simulink model "mpc_CSTR_PQ"  (R2017a)
settings: Solver=ode45  StartTime=0.0  StopTime=5  RelTol=1e-3
values from neighbouring files (symbols this model uses):
  Ap = [-1/(R*C)   1/C        0    -1/C      1/C        0 ... (first row only)    [GeneradoresInterconectados.m]
  Bp = [    0      0 ... (first row only)    [GeneradoresInterconectados.m]
  Cp = [    1      0 ... (first row only)    [GeneradoresInterconectados.m]
  Dp = zeros(2,2)    [GeneradoresInterconectados.m]
  I2 = 18    [GeneradoresInterconectados.m]
  Vabc = 160    [GeneradoresInterconectados.m]
undefined symbols (not defined in the file or in its folder): PI
libraries: powerlib_meascontrol x2, mpclib x1
settings Model: ExtModeTrigMode=oneshot  ExtModeArmWhenConnect=off  Creator=The MathWorks Inc.  LastModifiedBy=MarioAndres
settings DataIOCC: SaveFormat=Array  SaveOutput=off  SignalLogging=off  DSMLogging=off  SaveTime=off  SignalLoggingName=sigsOut
settings OptimizationCC: BooleanDataType=off  ExpressionDepthLimit=2147483647  InitFltsAndDblsToZero=on  LifeSpan=inf
settings DebuggingCC: SaveWithParameterizedLinksMsg=none  UnderspecifiedInitializationDetection=Classic  MergeDetectMultiDrivingBlocksExec=none  SignalResolutionControl=TryResolveAllWithWarning  MultiTaskDSMMsg=warning  MultiTaskCondExecSysMsg=none  IntegerOverflowMsg=none  FcnCallInpInsideContextMsg=warning  StateNameClashWarn=warning  SFUnexpectedBacktrackingDiag=warning  SFNoUnconditionalDefaultTransitionDiag=warning  SFExecutionAtInitializationDiag=none  IntegerSaturationMsg=none
settings HardwareCC: ProdBitPerPointer=32  ProdBitPerSizeT=32  ProdBitPerPtrDiffT=32  ProdLargestAtomicFloat=None  ProdIntDivRoundTo=Undefined  ProdEndianess=Unspecified  ProdWordSize=32  ProdHWDeviceType=32-bit Generic  TargetUnknown=on
settings ModelReferenceCC: PropagateSignalLabelsOutOfModel=off
settings GRTTargetCC: TargetFcnLib=ansi_tfl_tmw.mat  TargetLangStandard=C89/C90 (ANSI)  GeneratePreprocessorConditionals=Disable all  CombineOutputUpdateFcns=off  GRTInterface=on
settings ConfigComp: CovMetricSettings=dw  CovHtmlReporting=on  CovSaveCumulativeToWorkspaceVar=on  CovSaveSingleToWorkspaceVar=on  CovExternalEMLEnable=off  CovSFcnEnable=off

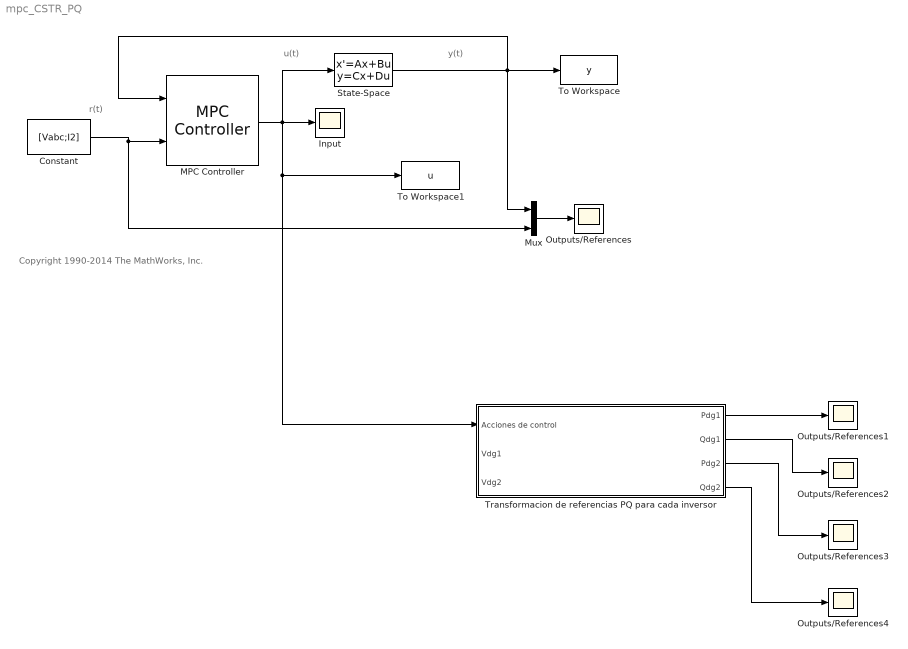
== system mpc_CSTR_PQ ==
  note: u(t)
  note: y(t)
  note: r(t)
  note: Copyright 1990-2014 The MathWorks, Inc.
  Constant : Constant  Value=[Vabc;I2]
  Input : Scope
  MPC Controller : mpclib/MPC Controller  mpcobj=mpcobj  x0=[]  is_multiple=0  enable_value=0  return_u0=off  ref_from_ws=off  ref_signal_name=[]  ref_preview=on  md_from_ws=off  md_signal_name=[]  md_preview=on  from_project=off  project_file=MPCtask.mat  md_inport=off  mv_inport=off  cost_outport=off  return_sequence=off  return_qpstatus=off  return_state=off  state_inport=off  lims_inport=off  ywt_inport=off  is_designfromscratch=0  uwt_inport=off  duwt_inport=off  rhoeps_inport=off  uref_inport=off  n_ts=0.1  n_mv=2  n_md=0  n_ud=0  n_mo=2  n_uo=0  BlockDataType=double  SampleTimeInherited=off  switch_inport=off
  Mux : Mux  Inputs=2
  Outputs/References{,1..4} (5 alike) : Scope
  State-Space : StateSpace  A=Ap  B=Bp  C=Cp  D=Dp  X0=0
  To Workspace : ToWorkspace  VariableName=y  SampleTime=-1
      settings: MaxDataPoints=Inf
  To Workspace1 : ToWorkspace  VariableName=u  SampleTime=-1
      settings: MaxDataPoints=Inf
  Transformacion de referencias PQ para cada inversor : Subsystem
  wires:
  MPC Controller/1 -> State-Space/1, Input/1, Transformacion de referencias PQ para cada inversor/1(Acciones de control), To Workspace1/1
  State-Space/1 -> To Workspace/1, Mux/1, MPC Controller/1
  Mux/1 -> Outputs/References/1
  Constant/1 -> Mux/2, MPC Controller/2
  Transformacion de referencias PQ para cada inversor/1(Pdg1) -> Outputs/References1/1
  Transformacion de referencias PQ para cada inversor/2(Qdg1) -> Outputs/References2/1
  Transformacion de referencias PQ para cada inversor/3(Pdg2) -> Outputs/References3/1
  Transformacion de referencias PQ para cada inversor/4(Qdg2) -> Outputs/References4/1

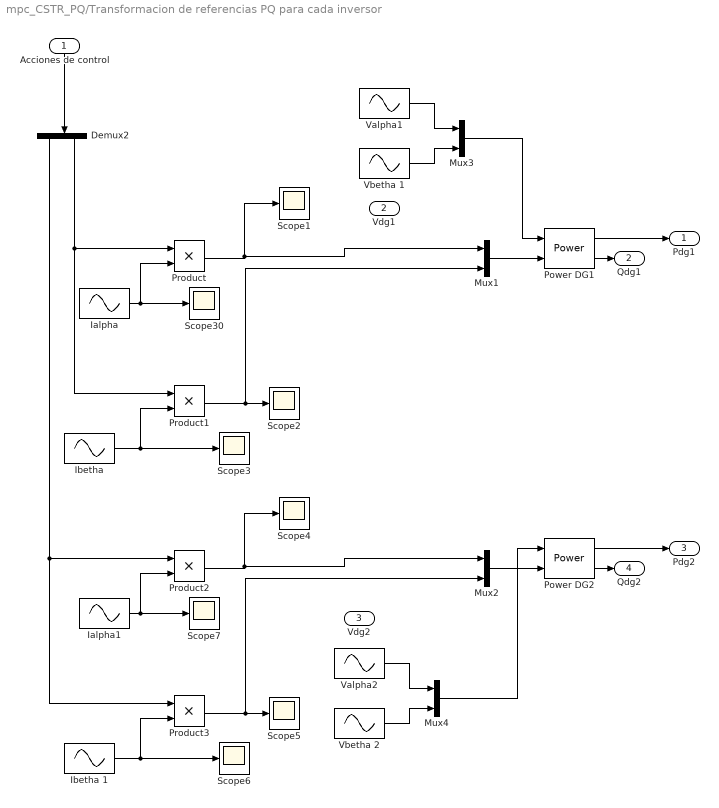
== system mpc_CSTR_PQ/Transformacion de referencias PQ para cada inversor ==
  Acciones de control : Inport
  Vdg1 : Inport  Port=2
  Vdg2 : Inport  Port=3
  Demux2 : Demux  Outputs=2
  Ialpha : Sin  Frequency=2*pi*60  Phase=pi/2  SampleTime=0.0001
  Ialpha1 : Sin  Frequency=2*pi*60  Phase=pi/2  SampleTime=0.0001
  "Ibetha " : Sin  Frequency=2*pi*60  SampleTime=0.0001
  Ibetha 1 : Sin  Frequency=2*pi*60  SampleTime=0.0001
  Mux{1..4} (4 alike) : Mux  Inputs=2
  Power DG1 : powerlib_meascontrol/Measurements/Power  Freq=60  Vinit=[1, 0]  Iinit=[1, 0]  Ts=0
      settings: SourceProductName=Simscape Power Systems
  Power DG2 : powerlib_meascontrol/Measurements/Power  Freq=60  Vinit=[1, 0]  Iinit=[1, 0]  Ts=0
      settings: SourceProductName=Simscape Power Systems
  Product{,1..3} (4 alike) : Product
  Scope{1..7,30} (8 alike) : Scope
  Valpha1 : Sin  Amplitude=120  Frequency=2*pi*60  Phase=pi/2  SampleTime=0.0001
  Valpha2 : Sin  Amplitude=120  Frequency=2*pi*60  Phase=pi/2  SampleTime=0.0001
  Vbetha 1 : Sin  Amplitude=120  Frequency=2*pi*60  Phase=PI/2  SampleTime=0.0001
  Vbetha 2 : Sin  Amplitude=120  Frequency=2*pi*60  SampleTime=0.0001
  Pdg1 : Outport
  Qdg1 : Outport  Port=2
  Pdg2 : Outport  Port=3
  Qdg2 : Outport  Port=4
  wires:
  Ialpha/1 -> Product/2, Scope30/1
  Mux1/1 -> Power DG1/2
  Power DG2/1 -> Pdg2/1
  Power DG2/2 -> Qdg2/1
  Power DG1/2 -> Qdg1/1
  Power DG1/1 -> Pdg1/1
  Mux2/1 -> Power DG2/2
  "Ibetha "/1 -> Product1/2, Scope3/1
  Product1/1 -> Mux1/2, Scope2/1
  Product/1 -> Mux1/1, Scope1/1
  Valpha1/1 -> Mux3/1
  Mux3/1 -> Power DG1/1
  Valpha2/1 -> Mux4/1
  Mux4/1 -> Power DG2/1
  Acciones de control/1 -> Demux2/1
  Demux2/2 -> Product1/1, Product/1
  Vbetha 1/1 -> Mux3/2
  Vbetha 2/1 -> Mux4/2
  Product2/1 -> Mux2/1, Scope4/1
  Ialpha1/1 -> Product2/2, Scope7/1
  Product3/1 -> Mux2/2, Scope5/1
  Demux2/1 -> Product2/1, Product3/1
  Ibetha 1/1 -> Product3/2, Scope6/1
